simulink library "Propulsion_Lib"  (R2016b)
settings: Solver=ode45  StartTime=0.0  StopTime=10.0  RelTol=1e-3
values from neighbouring files (symbols this model uses):
  AC =     [UAV_modelconfig.mat]
undefined symbols (not defined in the file or in its folder): TrimCondition
libraries: Propulsion_Lib x1, simulink x1, aerolibbdyn x1, aerolibtransform2 x1, UMNBlocks_Lib x1
settings Model: Creator=Paul Freeman  LastModifiedBy=UAVLAB
settings DataIOCC: LimitDataPoints=on  SaveFormat=Array  SignalLoggingSaveFormat=ModelDataLogs
settings OptimizationCC: BlockReduction=off  BooleanDataType=off  ExpressionDepthLimit=2147483647  LifeSpan=inf
settings DebuggingCC: SaveWithParameterizedLinksMsg=none  UnderspecifiedInitializationDetection=Classic  MergeDetectMultiDrivingBlocksExec=none  SignalResolutionControl=TryResolveAllWithWarning  FcnCallInpInsideContextMsg=warning  StateNameClashWarn=warning  StrictBusMsg=Warning  SFUnexpectedBacktrackingDiag=warning  SFNoUnconditionalDefaultTransitionDiag=warning  SFExecutionAtInitializationDiag=none
settings HardwareCC: ProdBitPerPointer=32  ProdBitPerSizeT=32  ProdBitPerPtrDiffT=32  ProdLargestAtomicFloat=None  ProdIntDivRoundTo=Undefined  ProdEndianess=Unspecified  ProdWordSize=32  ProdHWDeviceType=32-bit Generic  TargetUnknown=on
settings ModelReferenceCC: PropagateSignalLabelsOutOfModel=off
settings GRTTargetCC: TargetLangStandard=C89/C90 (ANSI)  GeneratePreprocessorConditionals=Disable all  CombineOutputUpdateFcns=off  GRTInterface=on
settings ConfigComp: CovMetricSettings=dw  CovHtmlReporting=on  CovSaveCumulativeToWorkspaceVar=on  CovSaveSingleToWorkspaceVar=on  CovExternalEMLEnable=off

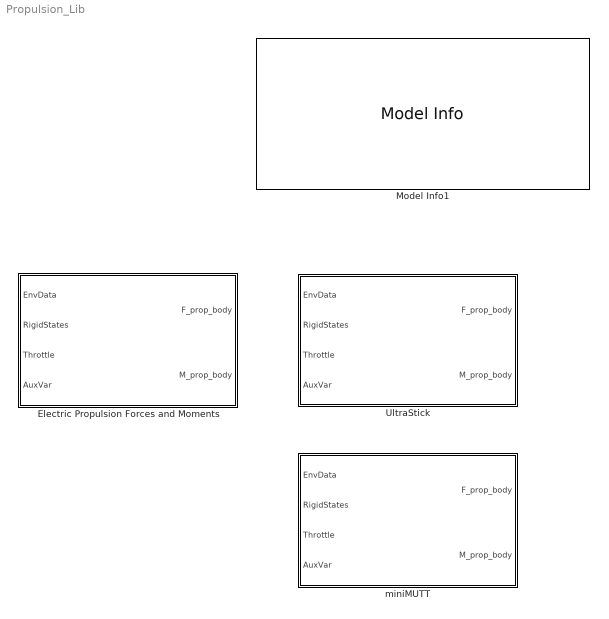
== system Propulsion_Lib ==
  Electric Propulsion Forces and Moments : Subsystem  BlockChoice=miniMUTT  mask{aircraft=AC.aircraft}
      mask prompts: aircraft "Aircraft type:"
      mask init:
      | pathname = gcb;
      | 
      | switch lower(aircraft)
      |     case 'ultrastick120'
      |         set_param(pathname,'BlockChoice','UltraStick');
      |     case 'ultrastick25e'
      |         set_param(pathname,'BlockChoice','UltraStick');
      |     case 'minimutt'
      |         set_param(pathname,'BlockChoice','miniMUTT');
      | end
      settings: TemplateBlock=self  MemberBlocks=UltraStick,miniMUTT
  Model Info1 : simulink/Model-Wide Utilities/Model Info  BlockCM=None  Frame=on  DisplayStringWithTags=|  HorizontalTextAlignment=Left  LeftAlignmentValue=0.02  SourceBlockDiagram=Propulsion_Lib  TagMaxNumber=20
      | MODEL INFORMATION
      | Propulsion Library
      | 
      | University of Minnesota
      | Aerospace Engineering and Mechanics
      | Copyright 2011 Regents of the University of Minnesota. All rights reserved.
      | 
      | == SVN Info ==
      | Last modified by %<LastModifiedBy> on %<LastModificationDate>
  UltraStick : Subsystem
  miniMUTT : Subsystem

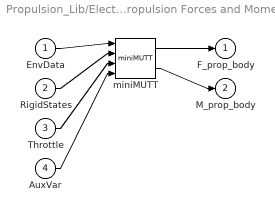
== system Propulsion_Lib/Electric Propulsion Forces and Moments ==
  EnvData : Inport
  RigidStates : Inport  Port=2
  Throttle : Inport  Port=3
  AuxVar : Inport  Port=4
  miniMUTT : Propulsion_Lib/miniMUTT
  F_prop_body : Outport
  M_prop_body : Outport  Port=2
  wires:
  EnvData/1 -> miniMUTT/1
  RigidStates/1 -> miniMUTT/2
  Throttle/1 -> miniMUTT/3
  AuxVar/1 -> miniMUTT/4
  miniMUTT/1 -> F_prop_body/1
  miniMUTT/2 -> M_prop_body/1

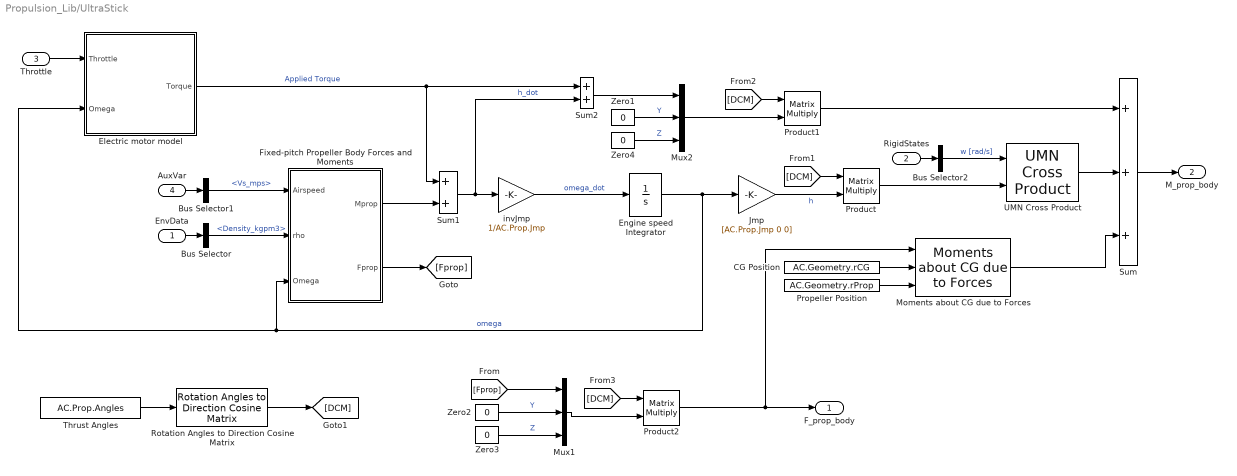
== system Propulsion_Lib/UltraStick ==
  EnvData : Inport  OutDataTypeStr=Bus: EnvData
  RigidStates : Inport  Port=2  OutDataTypeStr=Bus: RigidStates
  Throttle : Inport  Port=3  OutDataTypeStr=double
  AuxVar : Inport  Port=4  OutDataTypeStr=Bus: AuxVar
  Bus Selector : BusSelector  OutputSignals=Density_kgpm3
  Bus Selector1 : BusSelector  OutputSignals=WindAxesParams.Vs_mps
  Bus Selector2 : BusSelector  OutputSignals=AngVel.p_rps,AngVel.q_rps,AngVel.r_rps  OutputAsBus=on
  CG Position : Constant  Value=AC.Geometry.rCG
  Electric motor model : Subsystem
  Engine speed Integrator : Integrator  InitialCondition=TrimCondition.EngineSpeedIni  LimitOutput=on  UpperSaturationLimit=AC.Prop.OmegaSaturation.Upper  LowerSaturationLimit=AC.Prop.OmegaSaturation.Lower
  Fixed-pitch Propeller Body Forces and Moments : Subsystem
  Jmp : Gain  Gain=[AC.Prop.Jmp 0 0]  SaturateOnIntegerOverflow=on  OutDataTypeStr=Inherit: Same as input  ParamDataTypeStr=Inherit: Same as input
  Moments about CG due to Forces : aerolibbdyn/Moments about CG  due to Forces
  Mux1 : Mux  Inputs=3
  Mux2 : Mux  Inputs=3
  Product : Product  Multiplication=Matrix(*)  RndMeth=Zero
  Product1 : Product  Multiplication=Matrix(*)  RndMeth=Zero
  Product2 : Product  Multiplication=Matrix(*)  RndMeth=Zero
  Propeller Position : Constant  Value=AC.Geometry.rProp
  Rotation Angles to Direction Cosine Matrix : aerolibtransform2/Rotation Angles to Direction Cosine Matrix  rotationOrder=ZYX
  Sum : Sum  Inputs=+++
  Sum1 : Sum  SaturateOnIntegerOverflow=on  InputSameDT=on  OutDataTypeStr=Inherit: Same as first input
  Sum2 : Sum
  Thrust Angles : Constant  Value=AC.Prop.Angles
  UMN Cross Product : UMNBlocks_Lib/UMN Cross Product
  Zero{1..4} (4 alike) : Constant  Value=0
  invJmp : Gain  Gain=1/AC.Prop.Jmp
  F_prop_body : Outport
  M_prop_body : Outport  Port=2
  wires:
  Moments about CG due to Forces/1 -> Sum/3
  UMN Cross Product/1 -> Sum/2
  Product1/1 -> Sum/1
  Mux2/1 -> Product1/2
  Sum2/1 -> Mux2/1
  Zero1/1 -> Mux2/2  "Y"
  Zero4/1 -> Mux2/3  "Z"
  Product/1 -> UMN Cross Product/2
  Product2/1 -> F_prop_body/1, Moments about CG due to Forces/1
  Mux1/1 -> Product2/2
  [DCM] -> Product2/1
  [DCM] -> Product1/1
  [DCM] -> Product/1
  Rotation Angles to Direction Cosine Matrix/1 -> [DCM]
  Thrust Angles/1 -> Rotation Angles to Direction Cosine Matrix/1
  Bus Selector2/1 -> UMN Cross Product/1  "w [rad/s]"
  Jmp/1 -> Product/2  "h"
  Fixed-pitch Propeller Body Forces and Moments/2(Fprop) -> [Fprop]
  Fixed-pitch Propeller Body Forces and Moments/1(Mprop) -> Sum1/2
  Bus Selector/1 -> Fixed-pitch Propeller Body Forces and Moments/2(rho)  "<Density_kgpm3>"
  Bus Selector1/1 -> Fixed-pitch Propeller Body Forces and Moments/1(Airspeed)  "<Vs_mps>"
  [Fprop] -> Mux1/1
  RigidStates/1 -> Bus Selector2/1
  Sum/1 -> M_prop_body/1
  Propeller Position/1 -> Moments about CG due to Forces/3
  CG Position/1 -> Moments about CG due to Forces/2
  AuxVar/1 -> Bus Selector1/1
  EnvData/1 -> Bus Selector/1
  Zero2/1 -> Mux1/2  "Y"
  Zero3/1 -> Mux1/3  "Z"
  Engine speed Integrator/1 -> Jmp/1, Fixed-pitch Propeller Body Forces and Moments/3(Omega), Electric motor model/2(Omega)  "omega"
  Electric motor model/1(Torque) -> Sum2/1, Sum1/1  "Applied Torque"
  Throttle/1 -> Electric motor model/1(Throttle)
  Sum1/1 -> Sum2/2, invJmp/1  "h_dot"
  invJmp/1 -> Engine speed Integrator/1  "omega_dot"

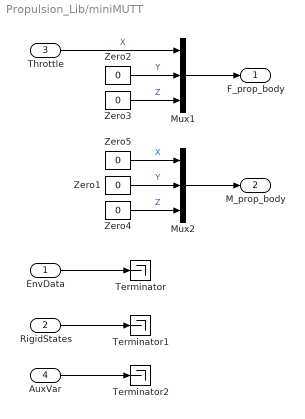
== system Propulsion_Lib/miniMUTT ==
  EnvData : Inport
  RigidStates : Inport  Port=2
  Throttle : Inport  Port=3  OutDataTypeStr=double
  AuxVar : Inport  Port=4
  Mux1 : Mux  Inputs=3
  Mux2 : Mux  Inputs=3
  Terminator : Terminator
  Terminator1 : Terminator
  Terminator2 : Terminator
  Zero{1..5} (5 alike) : Constant  Value=0
  F_prop_body : Outport
  M_prop_body : Outport  Port=2
  wires:
  Zero1/1 -> Mux2/2  "Y"
  Zero4/1 -> Mux2/3  "Z"
  Zero2/1 -> Mux1/2  "Y"
  Zero3/1 -> Mux1/3  "Z"
  Zero5/1 -> Mux2/1  "X"
  Mux2/1 -> M_prop_body/1
  Throttle/1 -> Mux1/1  "X"
  Mux1/1 -> F_prop_body/1
  EnvData/1 -> Terminator/1
  AuxVar/1 -> Terminator2/1
  RigidStates/1 -> Terminator1/1

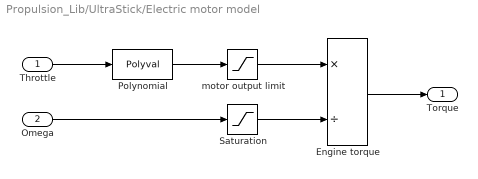
== system Propulsion_Lib/UltraStick/Electric motor model ==
  Throttle : Inport  OutDataTypeStr=double
  Omega : Inport  Port=2  OutDataTypeStr=double
  Engine torque : Product  Inputs=*/  SaturateOnIntegerOverflow=on  InputSameDT=on  OutDataTypeStr=Inherit: Same as first input
  Polynomial : Polyval  Coefs=AC.Prop.Power
  Saturation : Saturate  UpperLimit=AC.Prop.OmegaSaturation.Upper  LowerLimit=AC.Prop.OmegaSaturation.Lower
  motor output limit : Saturate  UpperLimit=AC.Prop.ThrottleOutputLimit.Upper  LowerLimit=AC.Prop.ThrottleOutputLimit.Lower
  Torque : Outport
  wires:
  motor output limit/1 -> Engine torque/1
  Throttle/1 -> Polynomial/1
  Polynomial/1 -> motor output limit/1
  Omega/1 -> Saturation/1
  Engine torque/1 -> Torque/1
  Saturation/1 -> Engine torque/2

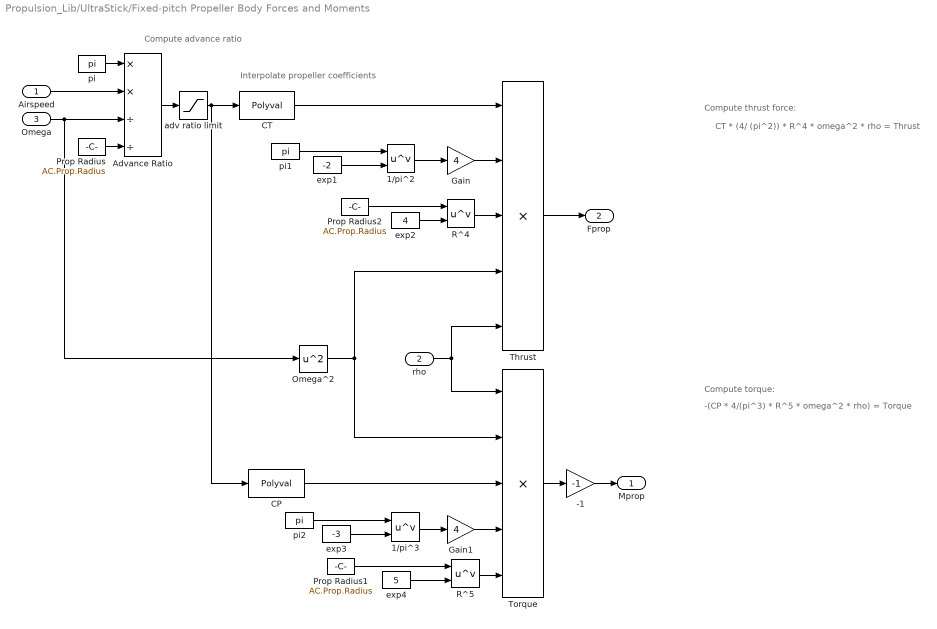
== system Propulsion_Lib/UltraStick/Fixed-pitch Propeller Body Forces and Moments ==
  note: -(CP * 4/(pi^3) * R^5 * omega^2 * rho) = Torque
  note: CT * (4/ (pi^2)) * R^4 * omega^2 * rho = Thrust
  note: Compute advance ratio
  note: Compute thrust force:
  note: Interpolate propeller coefficients
  note: Compute torque:
  Airspeed : Inport  OutDataTypeStr=double
  rho : Inport  Port=2  OutDataTypeStr=double
  Omega : Inport  Port=3  OutDataTypeStr=double
  -1 : Gain  Gain=-1  SaturateOnIntegerOverflow=on  OutDataTypeStr=Inherit: Same as input  ParamDataTypeStr=Inherit: Same as input
  1/pi^2 : Math  Operator=pow  SaturateOnIntegerOverflow=on
  1/pi^3 : Math  Operator=pow  SaturateOnIntegerOverflow=on
  Advance Ratio : Product  Inputs=**//  SaturateOnIntegerOverflow=on  InputSameDT=on  OutDataTypeStr=Inherit: Same as first input
  CP : Polyval  Coefs=AC.Prop.CP
  CT : Polyval  Coefs=AC.Prop.CT
  Gain : Gain  Gain=4  SaturateOnIntegerOverflow=on  OutDataTypeStr=Inherit: Same as input  ParamDataTypeStr=Inherit: Same as input
  Gain1 : Gain  Gain=4  SaturateOnIntegerOverflow=on  OutDataTypeStr=Inherit: Same as input  ParamDataTypeStr=Inherit: Same as input
  Omega^2 : Math  Operator=square  SaturateOnIntegerOverflow=on
  Prop Radius : Constant  Value=AC.Prop.Radius
  Prop Radius1 : Constant  Value=AC.Prop.Radius
  Prop Radius2 : Constant  Value=AC.Prop.Radius
  R^4 : Math  Operator=pow  SaturateOnIntegerOverflow=on
  R^5 : Math  Operator=pow  SaturateOnIntegerOverflow=on
  Thrust : Product  Inputs=5  SaturateOnIntegerOverflow=on  InputSameDT=on  OutDataTypeStr=Inherit: Same as first input
  Torque : Product  Inputs=5  SaturateOnIntegerOverflow=on  InputSameDT=on  OutDataTypeStr=Inherit: Same as first input
  adv ratio limit : Saturate  UpperLimit=0.7  LowerLimit=0
  exp1 : Constant  Value=-2
  exp2 : Constant  Value=4
  exp3 : Constant  Value=-3
  exp4 : Constant  Value=5
  pi : Constant  Value=pi
  pi1 : Constant  Value=pi
  pi2 : Constant  Value=pi
  Mprop : Outport
  Fprop : Outport  Port=2
  wires:
  adv ratio limit/1 -> CP/1, CT/1
  -1/1 -> Mprop/1
  pi/1 -> Advance Ratio/1
  pi2/1 -> 1/pi^3/1
  Prop Radius2/1 -> R^4/1
  Prop Radius1/1 -> R^5/1
  exp1/1 -> 1/pi^2/2
  Airspeed/1 -> Advance Ratio/2
  rho/1 -> Torque/1, Thrust/5
  Omega/1 -> Advance Ratio/3, Omega^2/1
  pi1/1 -> 1/pi^2/1
  Prop Radius/1 -> Advance Ratio/4
  Advance Ratio/1 -> adv ratio limit/1
  Omega^2/1 -> Torque/2, Thrust/4
  exp3/1 -> 1/pi^3/2
  1/pi^2/1 -> Gain/1
  1/pi^3/1 -> Gain1/1
  exp2/1 -> R^4/2
  R^4/1 -> Thrust/3
  exp4/1 -> R^5/2
  R^5/1 -> Torque/5
  Gain/1 -> Thrust/2
  Gain1/1 -> Torque/4
  Thrust/1 -> Fprop/1
  Torque/1 -> -1/1
  CT/1 -> Thrust/1
  CP/1 -> Torque/3
